simulink model "ADU_Integration_Y2016_simulation"  (R2016b)
settings: Solver=FixedStepDiscrete  StartTime=240  StopTime=300  FixedStep=0.01  RelTol=1e-3  EnableMultiTasking=on
PostLoadFcn:
  | , if any(exist('dsrtsu_mdlpostloadfcn', 'file') == [2, 3, 6]), try dsrtsu_mdlpostloadfcn('Execute', bdroot); catch fprintf('Error in PostLoadFcn (dsrtsu_mdlpostloadfcn) for model "%s":\n %s\n', bdroot, lasterr); end, end,
InitFcn:
  | load 'data/chi2_dat';
  | load 'data/innerLine_struct';
  | load 'data/middleLine_struct';
  | load 'data/outerLine_struct';
  | load 'data/innerLine';
  | load 'data/middleLine';
  | load 'data/outerLine';
  | load 'data/landmarks_patac_schimmel_ccw';
  | load 'data/patac_navi_array';
  | load 'data/sensor';
  | load 'data/map_struct';
  | addpath map_src
  | Integration_Parameter;
  | load 'TestData_001';
values from neighbouring files (symbols this model uses):
  TestData_001 =     [TestData_001.mat]
undefined symbols (not defined in the file or in its folder): a, chi2_dat, innerLine, landmarks_patac_schimmel_ccw, middleLine, outerLine, patac_navi_array, StartNum
libraries: simulink x36, rtican x1
(part 9 of 20)

== system ADU_Integration_Y2016_simulation/Fusion_Model/Fusion_Block/Side_Fusion/Side_Fusion/Tracker_Update.Tracker_Filter.Update.Update/Model_Update/Subsystem ==
  DataIn : Inport
  Constant : Constant  Value=[1;0;0;0]
  Constant1 : Constant  Value=[0;1;0;0]
  Constant2 : Constant  Value=[0;0;1;0]
  Constant3 : Constant  Value=[0;0;0;1]
  Demux{,1..4} (5 alike) : Demux
  PK_Cal : Subsystem
  Product{,1..3} (4 alike) : Product  Multiplication=Matrix(*)  RndMeth=Zero
  X_K_Cal : Subsystem
  RangeX : Outport
  VelX : Outport  Port=2
  RangeY : Outport  Port=3
  VelY : Outport  Port=4
  P11 : Outport  Port=5
  P12 : Outport  Port=6
  P13 : Outport  Port=7
  P14 : Outport  Port=8
  P21 : Outport  Port=9
  P22 : Outport  Port=10
  P23 : Outport  Port=11
  P24 : Outport  Port=12
  P31 : Outport  Port=13
  P32 : Outport  Port=14
  P33 : Outport  Port=15
  P34 : Outport  Port=16
  P41 : Outport  Port=17
  P42 : Outport  Port=18
  P43 : Outport  Port=19
  P44 : Outport  Port=20
  wires:
  X_K_Cal/1(X_K) -> Demux/1
  Constant/1 -> Product/2
  Product/1 -> Demux1/1
  Demux1/1 -> P11/1
  Demux1/2 -> P21/1
  Demux1/3 -> P31/1
  PK_Cal/1(P_K) -> Product3/1, Product2/1, Product/1, Product1/1
  Demux1/4 -> P41/1
  Constant1/1 -> Product1/2
  Product1/1 -> Demux2/1
  Demux2/1 -> P12/1
  Demux2/2 -> P22/1
  Demux2/3 -> P32/1
  Demux2/4 -> P42/1
  Constant2/1 -> Product2/2
  Product2/1 -> Demux3/1
  Demux3/1 -> P13/1
  Demux3/2 -> P23/1
  Demux3/3 -> P33/1
  Demux3/4 -> P43/1
  Constant3/1 -> Product3/2
  Product3/1 -> Demux4/1
  Demux4/1 -> P14/1
  Demux4/2 -> P24/1
  Demux4/3 -> P34/1
  Demux4/4 -> P44/1
  Demux/1 -> RangeX/1  "Range_X"
  Demux/2 -> VelX/1  "Velocity_X"
  Demux/3 -> RangeY/1  "Range_Y"
  Demux/4 -> VelY/1  "Velocity_Y"
  DataIn/1 -> X_K_Cal/1(DataIn), PK_Cal/1(DataIn)

== system ADU_Integration_Y2016_simulation/Fusion_Model/Fusion_Block/Side_Fusion/Side_Fusion/Tracker_Update.Tracker_Filter.Update.Update/Model_Update/Subsystem1 ==
  Pre_x : Inport
  Pre_vx : Inport  Port=2
  Pre_y : Inport  Port=3
  Pre_vy : Inport  Port=4
  pre_p11 : Inport  Port=5
  pre_p12 : Inport  Port=6
  pre_p13 : Inport  Port=7
  pre_p14 : Inport  Port=8
  pre_p21 : Inport  Port=9
  pre_p22 : Inport  Port=10
  pre_p23 : Inport  Port=11
  pre_p24 : Inport  Port=12
  pre_p31 : Inport  Port=13
  pre_p32 : Inport  Port=14
  pre_p33 : Inport  Port=15
  pre_p34 : Inport  Port=16
  pre_p41 : Inport  Port=17
  pre_p42 : Inport  Port=18
  pre_p43 : Inport  Port=19
  pre_p44 : Inport  Port=20
  mk : Inport  Port=21
  m00 : Inport  Port=22
  m01 : Inport  Port=23
  m2 : Inport  Port=24
  m10 : Inport  Port=25
  m11 : Inport  Port=26
  m12 : Inport  Port=27
  m20 : Inport  Port=28
  m21 : Inport  Port=29
  m22 : Inport  Port=30
  Pt0 : Inport  Port=31
  Bus Creator : BusCreator  Inputs=4
  Bus Creator1 : BusCreator  Inputs=6
  H : Constant  Value=[1 0 0 0;0 0 1 0]
  No_Zero1 : Subsystem
  No_Zero2 : Subsystem
  No_Zero3 : Subsystem
  No_Zero4 : Subsystem
  P_Gen : Subsystem
  Predict : Subsystem
  R11 : Constant  Value=0.7
  R12 : Constant  Value=0
  R21 : Constant  Value=0
  R22 : Constant  Value=0.8
  R_Cov_Gen : Subsystem
  Subsystem : Subsystem
  Source : Outport
  wires:
  H/1 -> Bus Creator1/1  "H[2X4]"
  R_Cov_Gen/1(Cov_R_Measuerment) -> Bus Creator1/2  "R[2X2]"
  Bus Creator1/1 -> Source/1
  Bus Creator/1 -> Predict/1(DataIn)  "Source"
  Pre_x/1 -> Bus Creator/1
  Pre_vy/1 -> Bus Creator/4
  Pre_y/1 -> Bus Creator/3
  Pre_vx/1 -> Bus Creator/2
  pre_p11/1 -> No_Zero1/1(In)
  pre_p12/1 -> P_Gen/2(pre_p12)
  pre_p13/1 -> P_Gen/3(pre_p13)
  pre_p14/1 -> P_Gen/4(pre_p14)
  pre_p21/1 -> P_Gen/5(pre_p21)
  pre_p22/1 -> No_Zero2/1(In)
  pre_p23/1 -> P_Gen/7(pre_p23)
  pre_p24/1 -> P_Gen/8(pre_p24)
  pre_p31/1 -> P_Gen/9(pre_p31)
  pre_p32/1 -> P_Gen/10(pre_p32)
  pre_p33/1 -> No_Zero3/1(In)
  pre_p34/1 -> P_Gen/12(pre_p34)
  pre_p41/1 -> P_Gen/13(pre_p41)
  pre_p42/1 -> P_Gen/14(pre_p42)
  pre_p43/1 -> P_Gen/15(pre_p43)
  pre_p44/1 -> No_Zero4/1(In)
  No_Zero1/1(Out) -> P_Gen/1(pre_p11)
  No_Zero2/1(Out) -> P_Gen/6(pre_p22)
  No_Zero3/1(Out) -> P_Gen/11(pre_p33)
  No_Zero4/1(Out) -> P_Gen/16(pre_p44)
  m22/1 -> Subsystem/10(m22)
  R21/1 -> R_Cov_Gen/3(R21)
  m21/1 -> Subsystem/9(m21)
  R12/1 -> R_Cov_Gen/2(R12)
  m00/1 -> Subsystem/2(m00)
  m2/1 -> Subsystem/4(m02)
  m10/1 -> Subsystem/5(m10)
  R22/1 -> R_Cov_Gen/4(R22)
  m12/1 -> Subsystem/7(m12)
  mk/1 -> Subsystem/1(mk)
  R11/1 -> R_Cov_Gen/1(R11)
  Predict/1(X_predit) -> Bus Creator1/3
  m01/1 -> Subsystem/3(m01)
  m20/1 -> Subsystem/8(m20)
  P_Gen/1(P_Pre[4x4]) -> Bus Creator1/4  "P[4X4]"
  m11/1 -> Subsystem/6(m11)
  Subsystem/1(Measurement) -> Bus Creator1/5
  Pt0/1 -> Bus Creator1/6  "Pt0"

== system ADU_Integration_Y2016_simulation/Fusion_Model/Fusion_Block/Global_Fusion/Fusion_Center/FusTrackPredict.Forecast/Predict/F/F_line_1 ==
  Data_in : Inport
  Bus Selector : BusSelector  OutputSignals=T
  Constant : Constant
  Constant1 : Constant  Value=0
  Constant2 : Constant  Value=[1;0;0;0]
  Constant3 : Constant  Value=0
  Math Function : Math  Operator=transpose  SaturateOnIntegerOverflow=on
  Mux : Mux
  Product : Product  Multiplication=Matrix(*)  RndMeth=Zero
  F_line_1 : Outport
  wires:
  Constant/1 -> Mux/1
  Constant1/1 -> Mux/4
  Data_in/1 -> Bus Selector/1
  Product/1 -> F_line_1/1
  Mux/1 -> Math Function/1
  Constant2/1 -> Product/1
  Math Function/1 -> Product/2
  Bus Selector/1 -> Mux/2  "<T>"
  Constant3/1 -> Mux/3

== system ADU_Integration_Y2016_simulation/Fusion_Model/Fusion_Block/Global_Fusion/Fusion_Center/FusTrackPredict.Forecast/Predict/F/F_line_2 ==
  Constant1 : Constant
  Constant3 : Constant  Value=0
  Constant4 : Constant  Value=0
  Constant5 : Constant  Value=[0;1;0;0]
  Constant6 : Constant  Value=0
  Math Function1 : Math  Operator=transpose  SaturateOnIntegerOverflow=on
  Mux1 : Mux
  Product1 : Product  Multiplication=Matrix(*)  RndMeth=Zero
  F_line_2 : Outport
  wires:
  Constant3/1 -> Mux1/1
  Constant4/1 -> Mux1/4
  Mux1/1 -> Math Function1/1
  Constant5/1 -> Product1/1
  Math Function1/1 -> Product1/2
  Constant1/1 -> Mux1/2
  Constant6/1 -> Mux1/3
  Product1/1 -> F_line_2/1

== system ADU_Integration_Y2016_simulation/Fusion_Model/Fusion_Block/Global_Fusion/Fusion_Center/FusTrackPredict.Forecast/Predict/F/F_line_3 ==
  Data_in : Inport
  Bus Selector : BusSelector  OutputSignals=T
  Constant : Constant
  Constant1 : Constant  Value=0
  Constant2 : Constant  Value=[0;0;1;0]
  Constant3 : Constant  Value=0
  Math Function : Math  Operator=transpose  SaturateOnIntegerOverflow=on
  Mux : Mux
  Product : Product  Multiplication=Matrix(*)  RndMeth=Zero
  F_line_3 : Outport
  wires:
  Product/1 -> F_line_3/1
  Constant3/1 -> Mux/1
  Bus Selector/1 -> Mux/4  "<T>"
  Mux/1 -> Math Function/1
  Constant2/1 -> Product/1
  Math Function/1 -> Product/2
  Constant/1 -> Mux/3
  Data_in/1 -> Bus Selector/1
  Constant1/1 -> Mux/2

== system ADU_Integration_Y2016_simulation/Fusion_Model/Fusion_Block/Global_Fusion/Fusion_Center/FusTrackPredict.Forecast/Predict/F/F_line_4 ==
  Constant1 : Constant  Value=0
  Constant3 : Constant  Value=0
  Constant4 : Constant
  Constant5 : Constant  Value=[0;0;0;1]
  Constant6 : Constant  Value=0
  Math Function1 : Math  Operator=transpose  SaturateOnIntegerOverflow=on
  Mux1 : Mux
  Product1 : Product  Multiplication=Matrix(*)  RndMeth=Zero
  F_line_4 : Outport
  wires:
  Product1/1 -> F_line_4/1
  Constant3/1 -> Mux1/1
  Constant4/1 -> Mux1/4
  Mux1/1 -> Math Function1/1
  Constant5/1 -> Product1/1
  Math Function1/1 -> Product1/2
  Constant1/1 -> Mux1/2
  Constant6/1 -> Mux1/3

== system ADU_Integration_Y2016_simulation/Fusion_Model/Fusion_Block/Side_Fusion/Side_Fusion/FusTrackPredict.Forecast/Predict/F/F_line_1 ==
  Data_in : Inport
  Bus Selector : BusSelector  OutputSignals=T
  Constant : Constant
  Constant1 : Constant  Value=0
  Constant2 : Constant  Value=[1;0;0;0]
  Constant3 : Constant  Value=0
  Math Function : Math  Operator=transpose  SaturateOnIntegerOverflow=on
  Mux : Mux
  Product : Product  Multiplication=Matrix(*)  RndMeth=Zero
  F_line_1 : Outport
  wires:
  Constant/1 -> Mux/1
  Constant1/1 -> Mux/4
  Data_in/1 -> Bus Selector/1
  Product/1 -> F_line_1/1
  Mux/1 -> Math Function/1
  Constant2/1 -> Product/1
  Math Function/1 -> Product/2
  Bus Selector/1 -> Mux/2  "<T>"
  Constant3/1 -> Mux/3

== system ADU_Integration_Y2016_simulation/Fusion_Model/Fusion_Block/Side_Fusion/Side_Fusion/FusTrackPredict.Forecast/Predict/F/F_line_2 ==
  Constant1 : Constant
  Constant3 : Constant  Value=0
  Constant4 : Constant  Value=0
  Constant5 : Constant  Value=[0;1;0;0]
  Constant6 : Constant  Value=0
  Math Function1 : Math  Operator=transpose  SaturateOnIntegerOverflow=on
  Mux1 : Mux
  Product1 : Product  Multiplication=Matrix(*)  RndMeth=Zero
  F_line_2 : Outport
  wires:
  Constant3/1 -> Mux1/1
  Constant4/1 -> Mux1/4
  Mux1/1 -> Math Function1/1
  Constant5/1 -> Product1/1
  Math Function1/1 -> Product1/2
  Constant1/1 -> Mux1/2
  Constant6/1 -> Mux1/3
  Product1/1 -> F_line_2/1

== system ADU_Integration_Y2016_simulation/Fusion_Model/Fusion_Block/Side_Fusion/Side_Fusion/FusTrackPredict.Forecast/Predict/F/F_line_3 ==
  Data_in : Inport
  Bus Selector : BusSelector  OutputSignals=T
  Constant : Constant
  Constant1 : Constant  Value=0
  Constant2 : Constant  Value=[0;0;1;0]
  Constant3 : Constant  Value=0
  Math Function : Math  Operator=transpose  SaturateOnIntegerOverflow=on
  Mux : Mux
  Product : Product  Multiplication=Matrix(*)  RndMeth=Zero
  F_line_3 : Outport
  wires:
  Product/1 -> F_line_3/1
  Constant3/1 -> Mux/1
  Bus Selector/1 -> Mux/4  "<T>"
  Mux/1 -> Math Function/1
  Constant2/1 -> Product/1
  Math Function/1 -> Product/2
  Constant/1 -> Mux/3
  Data_in/1 -> Bus Selector/1
  Constant1/1 -> Mux/2

== system ADU_Integration_Y2016_simulation/Fusion_Model/Fusion_Block/Side_Fusion/Side_Fusion/FusTrackPredict.Forecast/Predict/F/F_line_4 ==
  Constant1 : Constant  Value=0
  Constant3 : Constant  Value=0
  Constant4 : Constant
  Constant5 : Constant  Value=[0;0;0;1]
  Constant6 : Constant  Value=0
  Math Function1 : Math  Operator=transpose  SaturateOnIntegerOverflow=on
  Mux1 : Mux
  Product1 : Product  Multiplication=Matrix(*)  RndMeth=Zero
  F_line_4 : Outport
  wires:
  Product1/1 -> F_line_4/1
  Constant3/1 -> Mux1/1
  Constant4/1 -> Mux1/4
  Mux1/1 -> Math Function1/1
  Constant5/1 -> Product1/1
  Math Function1/1 -> Product1/2
  Constant1/1 -> Mux1/2
  Constant6/1 -> Mux1/3

== system ADU_Integration_Y2016_simulation/Fusion_Model/Fusion_Block/Side_Fusion/Side_Fusion/Tracker_Initial.cos_cal/Reltive_Deg_Cal/Side_Length_Cal/a_cal ==
  In1 : Inport
  Bus Selector2 : BusSelector  OutputSignals=x1,x2,y1,y2
  Math Function2 : Math  Operator=square  SaturateOnIntegerOverflow=on
  Math Function3 : Math  Operator=square  SaturateOnIntegerOverflow=on
  Sqrt : Sqrt  SaturateOnIntegerOverflow=on
  Subtract2 : Sum  Inputs=+-
  Subtract3 : Sum  Inputs=+-
  Subtract4 : Sum
  a : Outport
  wires:
  Subtract4/1 -> Sqrt/1
  Math Function2/1 -> Subtract4/1
  Sqrt/1 -> a/1
  Math Function3/1 -> Subtract4/2
  Bus Selector2/2 -> Subtract2/2  "<x2>"
  Subtract2/1 -> Math Function2/1
  Bus Selector2/3 -> Subtract3/1  "<y1>"
  Bus Selector2/4 -> Subtract3/2  "<y2>"
  Bus Selector2/1 -> Subtract2/1  "<x1>"
  In1/1 -> Bus Selector2/1
  Subtract3/1 -> Math Function3/1

== system ADU_Integration_Y2016_simulation/Fusion_Model/Fusion_Block/Side_Fusion/Side_Fusion/Tracker_Initial.cos_cal/Reltive_Deg_Cal/Side_Length_Cal/b_cal ==
  In1 : Inport
  Bus Selector2 : BusSelector  OutputSignals=x2,xm,y2,ym
  Math Function2 : Math  Operator=square  SaturateOnIntegerOverflow=on
  Math Function3 : Math  Operator=square  SaturateOnIntegerOverflow=on
  Sqrt : Sqrt  SaturateOnIntegerOverflow=on
  Subtract2 : Sum  Inputs=+-
  Subtract3 : Sum  Inputs=+-
  Subtract4 : Sum
  b : Outport
  wires:
  Subtract3/1 -> Math Function3/1
  In1/1 -> Bus Selector2/1
  Subtract2/1 -> Math Function2/1
  Math Function3/1 -> Subtract4/2
  Sqrt/1 -> b/1
  Math Function2/1 -> Subtract4/1
  Subtract4/1 -> Sqrt/1
  Bus Selector2/1 -> Subtract2/1  "<x2>"
  Bus Selector2/2 -> Subtract2/2  "<xm>"
  Bus Selector2/3 -> Subtract3/1  "<y2>"
  Bus Selector2/4 -> Subtract3/2  "<ym>"

== system ADU_Integration_Y2016_simulation/Fusion_Model/Fusion_Block/Side_Fusion/Side_Fusion/Tracker_Initial.cos_cal/Reltive_Deg_Cal/Side_Length_Cal/c_cal ==
  In1 : Inport
  Bus Selector2 : BusSelector  OutputSignals=xm,x1,ym,y1
  Math Function2 : Math  Operator=square  SaturateOnIntegerOverflow=on
  Math Function3 : Math  Operator=square  SaturateOnIntegerOverflow=on
  Sqrt : Sqrt  SaturateOnIntegerOverflow=on
  Subtract2 : Sum  Inputs=+-
  Subtract3 : Sum  Inputs=+-
  Subtract4 : Sum
  c : Outport
  wires:
  Subtract4/1 -> Sqrt/1
  Math Function2/1 -> Subtract4/1
  Sqrt/1 -> c/1
  Math Function3/1 -> Subtract4/2
  Subtract2/1 -> Math Function2/1
  In1/1 -> Bus Selector2/1
  Subtract3/1 -> Math Function3/1
  Bus Selector2/1 -> Subtract2/1  "<xm>"
  Bus Selector2/2 -> Subtract2/2  "<x1>"
  Bus Selector2/4 -> Subtract3/2  "<y1>"
  Bus Selector2/3 -> Subtract3/1  "<ym>"

== system ADU_Integration_Y2016_simulation/Fusion_Model/Fusion_Block/Side_Fusion/Side_Fusion/Tracker_Update.Tracker_Filter.Update.Update/Model_Update/Middle_Process/Kalman_Gain ==
  S : Inport
  Source : Inport  Port=2
  Bus Selector1 : BusSelector  OutputSignals=P[4X4],H[2X4]
  Divide : Product  Inputs=**/  Multiplication=Matrix(*)
  Math Function1 : Math  Operator=transpose  SaturateOnIntegerOverflow=on
  K : Outport
  wires:
  Divide/1 -> K/1  "K[4X2]"
  Source/1 -> Bus Selector1/1
  Bus Selector1/1 -> Divide/1  "<P[4X4]>"
  Bus Selector1/2 -> Math Function1/1  "<H[2X4]>"
  Math Function1/1 -> Divide/2  "[4X2]"
  S/1 -> Divide/3  "S[2x2]"

== system ADU_Integration_Y2016_simulation/Fusion_Model/Fusion_Block/Side_Fusion/Side_Fusion/Tracker_Update.Tracker_Filter.Update.Update/Model_Update/Middle_Process/S_Cal ==
  Source : Inport
  Bus Selector2 : BusSelector  OutputSignals=H[2X4],P[4X4],H[2X4],R[2X2]
  Math Function : Math  Operator=transpose  SaturateOnIntegerOverflow=on
  Product4 : Product  Inputs=3  Multiplication=Matrix(*)  RndMeth=Zero
  Subtract2 : Sum
  S : Outport
  wires:
  Bus Selector2/4 -> Subtract2/2  "<R[2X2]>"
  Math Function/1 -> Product4/3  "HT[4x2]"
  Subtract2/1 -> S/1  "S[2x2]"
  Bus Selector2/1 -> Product4/1  "<H[2X4]>"
  Bus Selector2/3 -> Math Function/1  "<H[2X4]>"
  Source/1 -> Bus Selector2/1
  Bus Selector2/2 -> Product4/2  "<P[4X4]>"
  Product4/1 -> Subtract2/1

== system ADU_Integration_Y2016_simulation/Fusion_Model/Fusion_Block/Side_Fusion/Side_Fusion/Tracker_Update.Tracker_Filter.Update.Update/Model_Update/Middle_Process/Subsystem ==
  Source : Inport
  Bus Creator1 : BusCreator  Inputs=2
  Bus Creator2 : BusCreator  Inputs=2
  Bus Creator3 : BusCreator  Inputs=2
  Bus Creator5 : BusCreator  Inputs=3
  Bus Selector1 : BusSelector  OutputSignals=Measurement.Measurement_2.Measurement_2_Possible,Measurement.Measurement_2.Measurement_2_X_Error,Measurement.Measurement_2.Measurement_2_Y_Error
  Bus Selector2 : BusSelector  OutputSignals=Measurement.Measurement_1.Measurement_1_Possible,Measurement.Measurement_1.Measurement_1_X_Error,Measurement.Measurement_1.Measurement_1_Y_Error
  Bus Selector3 : BusSelector  OutputSignals=Measurement.Measurement_3.Measurement_3_Possible,Measurement.Measurement_3.Measurement_3_X_Error,Measurement.Measurement_3.Measurement_3_Y_Error
  Mux : Mux  Inputs=2
  Mux1 : Mux  Inputs=2
  Mux2 : Mux  Inputs=2
  V_Cal : Subsystem
  MeasureData : Outport
  V : Outport  Port=2
  wires:
  Bus Selector3/1 -> Bus Creator3/1  "<Measurement_3_Possible>"
  Bus Creator5/1 -> V_Cal/1(In1), MeasureData/1
  Mux2/1 -> Bus Creator3/2  "Vt3[2X1]"
  Bus Selector3/3 -> Mux2/2  "<Measurement_3_Y_Error>"
  Bus Creator2/1 -> Bus Creator5/2  "Measure2"
  Bus Creator3/1 -> Bus Creator5/3  "Measure3"
  Bus Selector1/2 -> Mux1/1  "<Measurement_2_X_Error>"
  Mux1/1 -> Bus Creator2/2  "Vt2[2X1]"
  Bus Selector1/3 -> Mux1/2  "<Measurement_2_Y_Error>"
  Bus Selector1/1 -> Bus Creator2/1  "<Measurement_2_Possible>"
  Bus Selector3/2 -> Mux2/1  "<Measurement_3_X_Error>"
  Bus Creator1/1 -> Bus Creator5/1  "Measure1"
  Source/1 -> Bus Selector3/1, Bus Selector1/1, Bus Selector2/1
  Mux/1 -> Bus Creator1/2  "Vt1[2X1]"
  Bus Selector2/3 -> Mux/2  "<Measurement_1_Y_Error>"
  Bus Selector2/1 -> Bus Creator1/1  "<Measurement_1_Possible>"
  Bus Selector2/2 -> Mux/1  "<Measurement_1_X_Error>"
  V_Cal/1(V) -> V/1

== system ADU_Integration_Y2016_simulation/Fusion_Model/Fusion_Block/Side_Fusion/Side_Fusion/Tracker_Update.Tracker_Filter.Update.Update/Model_Update/Subsystem/PK_Cal ==
  DataIn : Inport
  P_Cal_1 : Subsystem
  P_Cal_2 : Subsystem
  P_Cal_3 : Subsystem
  Subtract1 : Sum  Inputs=+++
  P_K : Outport
  wires:
  DataIn/1 -> P_Cal_3/1(DataIn), P_Cal_2/1(DataIn), P_Cal_1/1(DataIn)
  P_Cal_3/1(DataOut) -> Subtract1/3
  Subtract1/1 -> P_K/1
  P_Cal_2/1(DataOut) -> Subtract1/2
  P_Cal_1/1(Data_Out) -> Subtract1/1

== system ADU_Integration_Y2016_simulation/Fusion_Model/Fusion_Block/Side_Fusion/Side_Fusion/Tracker_Update.Tracker_Filter.Update.Update/Model_Update/Subsystem/X_K_Cal ==
  DataIn : Inport
  Bus Selector2 : BusSelector  OutputSignals=Source.X_k[4X1],K[4X2],V[2X1]
  Divide3 : Product  Inputs=**  Multiplication=Matrix(*)
  Subtract1 : Sum
  X_K : Outport
  wires:
  DataIn/1 -> Bus Selector2/1
  Bus Selector2/2 -> Divide3/1  "<K[4X2]>"
  Divide3/1 -> Subtract1/2  "[4X1]"
  Bus Selector2/1 -> Subtract1/1  "<X_k[4X1]>"
  Subtract1/1 -> X_K/1
  Bus Selector2/3 -> Divide3/2  "<V[2X1]>"

== system ADU_Integration_Y2016_simulation/Fusion_Model/Fusion_Block/Side_Fusion/Side_Fusion/Tracker_Update.Tracker_Filter.Update.Update/Model_Update/Subsystem1/No_Zero1 ==
  In : Inport
  Abs : Abs
  Compare To Constant : simulink/Logic and Bit Operations/Compare To Constant  relop=>=  const=0.001  OutDataTypeStr=uint8
  Constant : Constant  Value=0.001
  Switch : Switch  Threshold=0.5
  Out : Outport
  wires:
  Constant/1 -> Switch/3
  Switch/1 -> Out/1
  Compare To Constant/1 -> Switch/2
  In/1 -> Switch/1, Abs/1
  Abs/1 -> Compare To Constant/1

== system ADU_Integration_Y2016_simulation/Fusion_Model/Fusion_Block/Side_Fusion/Side_Fusion/Tracker_Update.Tracker_Filter.Update.Update/Model_Update/Subsystem1/No_Zero2 ==
  In : Inport
  Abs : Abs
  Compare To Constant : simulink/Logic and Bit Operations/Compare To Constant  relop=>=  const=0.001  OutDataTypeStr=uint8
  Constant : Constant  Value=0.001
  Switch : Switch  Threshold=0.5
  Out : Outport
  wires:
  Abs/1 -> Compare To Constant/1
  In/1 -> Abs/1, Switch/1
  Compare To Constant/1 -> Switch/2
  Switch/1 -> Out/1
  Constant/1 -> Switch/3

== system ADU_Integration_Y2016_simulation/Fusion_Model/Fusion_Block/Side_Fusion/Side_Fusion/Tracker_Update.Tracker_Filter.Update.Update/Model_Update/Subsystem1/No_Zero3 ==
  In : Inport
  Abs : Abs
  Compare To Constant : simulink/Logic and Bit Operations/Compare To Constant  relop=>=  const=0.001  OutDataTypeStr=uint8
  Constant : Constant  Value=0.001
  Switch : Switch  Threshold=0.5
  Out : Outport
  wires:
  Constant/1 -> Switch/3
  Switch/1 -> Out/1
  Compare To Constant/1 -> Switch/2
  In/1 -> Switch/1, Abs/1
  Abs/1 -> Compare To Constant/1

== system ADU_Integration_Y2016_simulation/Fusion_Model/Fusion_Block/Side_Fusion/Side_Fusion/Tracker_Update.Tracker_Filter.Update.Update/Model_Update/Subsystem1/No_Zero4 ==
  In : Inport
  Abs : Abs
  Compare To Constant : simulink/Logic and Bit Operations/Compare To Constant  relop=>=  const=0.001  OutDataTypeStr=uint8
  Constant : Constant  Value=0.001
  Switch : Switch  Threshold=0.5
  Out : Outport
  wires:
  Abs/1 -> Compare To Constant/1
  In/1 -> Abs/1, Switch/1
  Compare To Constant/1 -> Switch/2
  Switch/1 -> Out/1
  Constant/1 -> Switch/3

== system ADU_Integration_Y2016_simulation/Fusion_Model/Fusion_Block/Side_Fusion/Side_Fusion/Tracker_Update.Tracker_Filter.Update.Update/Model_Update/Subsystem1/P_Gen ==
  pre_p11 : Inport
  pre_p12 : Inport  Port=2
  pre_p13 : Inport  Port=3
  pre_p14 : Inport  Port=4
  pre_p21 : Inport  Port=5
  pre_p22 : Inport  Port=6
  pre_p23 : Inport  Port=7
  pre_p24 : Inport  Port=8
  pre_p31 : Inport  Port=9
  pre_p32 : Inport  Port=10
  pre_p33 : Inport  Port=11
  pre_p34 : Inport  Port=12
  pre_p41 : Inport  Port=13
  pre_p42 : Inport  Port=14
  pre_p43 : Inport  Port=15
  pre_p44 : Inport  Port=16
  Add : Sum  Inputs=++++
  Gain : Gain  Gain=[1;0;0;0]  Multiplication=Matrix(K*u)
  Gain1 : Gain  Gain=[0;1;0;0]  Multiplication=Matrix(K*u)
  Gain2 : Gain  Gain=[0;0;1;0]  Multiplication=Matrix(K*u)
  Gain3 : Gain  Gain=[0;0;0;1]  Multiplication=Matrix(K*u)
  Math Function{1..4} (4 alike) : Math  Operator=transpose  SaturateOnIntegerOverflow=on
  Mux{,1..3} (4 alike) : Mux
  P_Pre[4x4] : Outport
  wires:
  Mux/1 -> Math Function2/1
  Math Function2/1 -> Gain/1
  Mux1/1 -> Math Function1/1
  Math Function1/1 -> Gain1/1
  Mux2/1 -> Math Function4/1
  Math Function4/1 -> Gain2/1
  Mux3/1 -> Math Function3/1
  Math Function3/1 -> Gain3/1
  Gain/1 -> Add/1
  Gain1/1 -> Add/2
  Gain2/1 -> Add/3
  Gain3/1 -> Add/4
  pre_p11/1 -> Mux/1
  pre_p12/1 -> Mux/2
  pre_p13/1 -> Mux/3
  pre_p14/1 -> Mux/4
  pre_p21/1 -> Mux1/1
  pre_p22/1 -> Mux1/2
  pre_p23/1 -> Mux1/3
  pre_p24/1 -> Mux1/4
  pre_p31/1 -> Mux2/1
  pre_p32/1 -> Mux2/2
  pre_p33/1 -> Mux2/3
  pre_p34/1 -> Mux2/4
  pre_p41/1 -> Mux3/1
  pre_p42/1 -> Mux3/2
  pre_p43/1 -> Mux3/3
  pre_p44/1 -> Mux3/4
  Add/1 -> P_Pre[4x4]/1

== system ADU_Integration_Y2016_simulation/Fusion_Model/Fusion_Block/Side_Fusion/Side_Fusion/Tracker_Update.Tracker_Filter.Update.Update/Model_Update/Subsystem1/Predict ==
  DataIn : Inport
  State_Predit : Subsystem
  X_predit : Outport
  wires:
  DataIn/1 -> State_Predit/1(Source)
  State_Predit/1(X_k) -> X_predit/1  "X_k[4X1]"

== system ADU_Integration_Y2016_simulation/Fusion_Model/Fusion_Block/Side_Fusion/Side_Fusion/Tracker_Update.Tracker_Filter.Update.Update/Model_Update/Subsystem1/R_Cov_Gen ==
  R11 : Inport
  R12 : Inport  Port=2
  R21 : Inport  Port=3
  R22 : Inport  Port=4
  Add : Sum
  Gain : Gain  Gain=[1;0]  Multiplication=Matrix(K*u)
  Gain1 : Gain  Gain=[0;1]  Multiplication=Matrix(K*u)
  Math Function1 : Math  Operator=transpose  SaturateOnIntegerOverflow=on
  Math Function2 : Math  Operator=transpose  SaturateOnIntegerOverflow=on
  Mux : Mux  Inputs=2
  Mux1 : Mux  Inputs=2
  Cov_R_Measuerment : Outport
  wires:
  Add/1 -> Cov_R_Measuerment/1
  R22/1 -> Mux1/2
  R21/1 -> Mux1/1
  R12/1 -> Mux/2
  R11/1 -> Mux/1
  Gain1/1 -> Add/2
  Gain/1 -> Add/1
  Math Function1/1 -> Gain1/1
  Mux1/1 -> Math Function1/1
  Math Function2/1 -> Gain/1
  Mux/1 -> Math Function2/1

== system ADU_Integration_Y2016_simulation/Fusion_Model/Fusion_Block/Side_Fusion/Side_Fusion/Tracker_Update.Tracker_Filter.Update.Update/Model_Update/Subsystem1/Subsystem ==
  mk : Inport
  m00 : Inport  Port=2
  m01 : Inport  Port=3
  m02 : Inport  Port=4
  m10 : Inport  Port=5
  m11 : Inport  Port=6
  m12 : Inport  Port=7
  m20 : Inport  Port=8
  m21 : Inport  Port=9
  m22 : Inport  Port=10
  Bus Creator1 : BusCreator  Inputs=3
  Bus Creator2 : BusCreator  Inputs=3
  Bus Creator3 : BusCreator  Inputs=3
  Bus Creator4 : BusCreator  Inputs=4
  Measurement : Outport
  wires:
  Bus Creator4/1 -> Measurement/1  "Measurement"
  m00/1 -> Bus Creator1/1
  m12/1 -> Bus Creator2/3
  m10/1 -> Bus Creator2/1
  m22/1 -> Bus Creator3/3
  m11/1 -> Bus Creator2/2
  m02/1 -> Bus Creator1/3
  m01/1 -> Bus Creator1/2
  Bus Creator2/1 -> Bus Creator4/2  "Measurement_2"
  m21/1 -> Bus Creator3/2
  m20/1 -> Bus Creator3/1
  mk/1 -> Bus Creator4/4
  Bus Creator1/1 -> Bus Creator4/1  "Measurement_1"
  Bus Creator3/1 -> Bus Creator4/3  "Measurement_3"

== system ADU_Integration_Y2016_simulation/Fusion_Model/Fusion_Block/Side_Fusion/Side_Fusion/Tracker_Update.Tracker_Filter.Update.Update/Model_Update/Middle_Process/Subsystem/V_Cal ==
  In1 : Inport
  Bus Selector4 : BusSelector  OutputSignals=Measure1.Measurement_1_Possible,Measure1.Vt1[2X1],Measure2.Measurement_2_Possible,Measure2.Vt2[2X1],Measure3.Measurement_3_Possible,Measure3.Vt3[2X1]
  Divide : Product  Inputs=**
  Divide1 : Product  Inputs=**
  Divide2 : Product  Inputs=**
  Subtract2 : Sum  Inputs=+++
  V : Outport
  wires:
  Divide/1 -> Subtract2/3
  Divide2/1 -> Subtract2/1
  Bus Selector4/4 -> Divide1/2  "<Vt2[2X1]>"
  Bus Selector4/5 -> Divide/1  "<Measurement_3_Possible>"
  Bus Selector4/2 -> Divide2/2  "<Vt1[2X1]>"
  In1/1 -> Bus Selector4/1
  Subtract2/1 -> V/1  "V[2X1]"
  Divide1/1 -> Subtract2/2
  Bus Selector4/3 -> Divide1/1  "<Measurement_2_Possible>"
  Bus Selector4/6 -> Divide/2  "<Vt3[2X1]>"
  Bus Selector4/1 -> Divide2/1  "<Measurement_1_Possible>"

== system ADU_Integration_Y2016_simulation/Fusion_Model/Fusion_Block/Side_Fusion/Side_Fusion/Tracker_Update.Tracker_Filter.Update.Update/Model_Update/Subsystem/PK_Cal/P_Cal_1 ==
  DataIn : Inport
  Bus Selector2 : BusSelector  OutputSignals=K[4X2],MeasureGen.Measure1.Measurement_1_Possible,MeasureGen.Measure1.Vt1[2X1],MeasureGen.Measure1.Vt1[2X1],MeasureGen.Measure2.Measurement_2_Possible,MeasureGen.Measure2.Vt2[2X1],MeasureGen.Measure2.Vt2[2X1],MeasureGen.Measure3.Measurement_3_Possible,MeasureGen.Measure3.Vt3[2X1],MeasureGen.Measure3.Vt3[2X1],V[2X1],V[2X1],K[4X2]
  Divide1 : Product  Inputs=**
  Divide2 : Product  Inputs=**
  Divide{3..4,6..7} (4 alike) : Product  Inputs=**  Multiplication=Matrix(*)
  Divide5 : Product  Inputs=**
  Divide8 : Product  Inputs=***  Multiplication=Matrix(*)
  Math Function{1..5} (5 alike) : Math  Operator=transpose  SaturateOnIntegerOverflow=on
  Subtract1 : Sum  Inputs=+-
  Subtract2 : Sum  Inputs=+++
  Data_Out : Outport
  wires:
  Subtract2/1 -> Subtract1/1  "[2X2]"
  Divide3/1 -> Divide1/2  "[2X2]"
  Bus Selector2/4 -> Math Function1/1  "<Vt1[2X1]>"
  Math Function1/1 -> Divide3/2  "[1X2]"
  Bus Selector2/7 -> Math Function2/1  "<Vt2[2X1]>"
  Bus Selector2/10 -> Math Function3/1  "<Vt3[2X1]>"
  Bus Selector2/3 -> Divide3/1  "<Vt1[2X1]>"
  Bus Selector2/2 -> Divide1/1  "<Measurement_1_Possible>"
  Bus Selector2/6 -> Divide4/1  "<Vt2[2X1]>"
  Divide4/1 -> Divide2/2  "[2X2]"
  Bus Selector2/12 -> Math Function4/1  "<V[2X1]>"
  Bus Selector2/5 -> Divide2/1  "<Measurement_2_Possible>"
  Math Function2/1 -> Divide4/2  "[1X2]"
  Math Function4/1 -> Divide7/2  "[1X2]"
  Divide5/1 -> Subtract2/3
  Subtract1/1 -> Divide8/2  "[2X2]"
  Math Function3/1 -> Divide6/2  "[1X2]"
  Divide7/1 -> Subtract1/2  "[2X2]"
  Divide2/1 -> Subtract2/2
  Bus Selector2/9 -> Divide6/1  "<Vt3[2X1]>"
  Bus Selector2/8 -> Divide5/1  "<Measurement_3_Possible>"
  Divide6/1 -> Divide5/2  "[2X2]"
  DataIn/1 -> Bus Selector2/1
  Bus Selector2/11 -> Divide7/1  "<V[2X1]>"
  Divide1/1 -> Subtract2/1
  Bus Selector2/13 -> Math Function5/1  "<K[4X2]>"
  Math Function5/1 -> Divide8/3  "[2X4]"
  Bus Selector2/1 -> Divide8/1  "<K[4X2]>"
  Divide8/1 -> Data_Out/1  "[4X4]"

== system ADU_Integration_Y2016_simulation/Fusion_Model/Fusion_Block/Side_Fusion/Side_Fusion/Tracker_Update.Tracker_Filter.Update.Update/Model_Update/Subsystem/PK_Cal/P_Cal_2 ==
  DataIn : Inport
  Bus Selector2 : BusSelector  OutputSignals=Source.Pt0,Source.P[4X4]
  Divide8 : Product  Inputs=**
  DataOut : Outport
  wires:
  Bus Selector2/1 -> Divide8/1  "<Pt0>"
  Bus Selector2/2 -> Divide8/2  "<P[4X4]>"
  DataIn/1 -> Bus Selector2/1
  Divide8/1 -> DataOut/1  "[4X4]"

== system ADU_Integration_Y2016_simulation/Fusion_Model/Fusion_Block/Side_Fusion/Side_Fusion/Tracker_Update.Tracker_Filter.Update.Update/Model_Update/Subsystem/PK_Cal/P_Cal_3 ==
  DataIn : Inport
  Bus Selector1 : BusSelector  OutputSignals=Source.Pt0,K[4X2],Source.H[2X4],Source.P[4X4]
  Constant_1 : Constant
  Divide1 : Product  Inputs=**  Multiplication=Matrix(*)
  Divide2 : Product  Inputs=**  Multiplication=Matrix(*)
  Divide3 : Product  Inputs=**
  I : Constant  Value=[1 0 0 0;0 1 0 0;0 0 1 0;0 0 0 1]
  Subtract1 : Sum  Inputs=+-
  Subtract2 : Sum  Inputs=+-
  DataOut : Outport
  wires:
  Bus Selector1/1 -> Subtract1/2  "<Pt0>"
  Bus Selector1/2 -> Divide1/1  "<K[4X2]>"
  Divide2/1 -> Divide3/2  "[4X4]"
  Divide1/1 -> Subtract2/2  "[4X4]"
  Bus Selector1/3 -> Divide1/2  "<H[2X4]>"
  Constant_1/1 -> Subtract1/1
  Divide3/1 -> DataOut/1  "[4X4]"
  I/1 -> Subtract2/1
  Subtract2/1 -> Divide2/1  "[4x4]"
  Bus Selector1/4 -> Divide2/2  "<P[4X4]>"
  Subtract1/1 -> Divide3/1
  DataIn/1 -> Bus Selector1/1

== system ADU_Integration_Y2016_simulation/Fusion_Model/Fusion_Block/Side_Fusion/Side_Fusion/Tracker_Update.Tracker_Filter.Update.Update/Model_Update/Subsystem1/Predict/State_Predit ==
  Source : Inport
  Bus Selector : BusSelector  OutputSignals=Pre_x,Pre_vx,Pre_y,Pre_vy
  Mux : Mux
  X_k : Outport
  wires:
  Source/1 -> Bus Selector/1
  Mux/1 -> X_k/1
  Bus Selector/1 -> Mux/1  "<Pre_x>"
  Bus Selector/3 -> Mux/3  "<Pre_y>"
  Bus Selector/4 -> Mux/4  "<Pre_vy>"
  Bus Selector/2 -> Mux/2  "<Pre_vx>"

== stateflow chart ADU_Integration_Y2016_simulation/Fusion_Model/Fusion_Block/Global_Fusion/ESR_TemporalAlig ==
  state [rangeX,rangeY]=TemporalAligFront(range,azimuth,W,L,InstallAngESR) [function]
  (default) -> (junction 95) : {
      | k=0;
      | ESR_Output=0;
      | }
  (junction 95) -> (junction 98) [order 1] : [k<64]
  (junction 98) -> (junction 104) [order 1] : [ESR_Input[k][0]!=0]
  (junction 101) -> (junction 95) : {
      | k++;
      | }
  (junction 95) -> (junction 96) [order 2]
  (junction 98) -> (junction 101) [order 2]
  (junction 104) -> (junction 106) : {
      | ESR_Output[k][0]=ESR_Input[k][0];%Target ID
      | [ESR_Output[k][1],ESR_Output[k][2]]=TemporalAligFront(ESR_Input[k][1],ESR_Input[k][2],W,L,0);
      | ESR_Output[k][3]=ESR_Input[k][3]; %Target DynamicMode
      | }
  (junction 106) -> (junction 101)
  (junction 96) -> (junction 158)
  (junction 158) -> (junction 160) [order 1] : [RollCount<=3]
  (junction 158) -> (junction 164) [order 2] : {
      | RollCount=0;
      | }
  (junction 160) -> (junction 163) : {
      | RollCount++;
      | }
  (junction 163) -> (junction 164)
  (junction 164) -> (junction 165)
  data: range function_input; rangeX function_output; rangeY function_output; azimuth function_input; W function_input double size=1; L function_input double size=1; InstallAngESR function_input double size=1; ESR_Input input double size=[64 4]; ESR_Output output double size=[64 4]; k local double size=1 =0; L constant double =5.2; W constant double =1.8; RollCount output double
  events: ESR_Trig input EITHER_EDGE_EVENT
